simulink model "ExampleOrientationOnCar"  (Simulink 9.2)
settings: Solver=FixedStepDiscrete  StartTime=0.0  StopTime=inf  FixedStep=TIMESTEP  RelTol=1e-3  EnableMultiTasking=on
PostLoadFcn:
  | TIMESTEP = 0.001;
  | 
  | gCGHeight = 0.3545;            % height of the car body reference point above the ground
  | gLeftWheelBase = 3.105;      % distance between left front and rear axles
  | CG_OFFSET_FROM_NOSE = [-gLeftWheelBase/2, 0, gCGHeight];
libraries: simulink x6, rFproPhysicsLib x4
settings Model: Creator=enewton  LastModifiedBy=SeanKavanagh
settings OptimizationCC: ExpressionDepthLimit=2147483647  EfficientFloat2IntCast=on
settings DebuggingCC: SolverPrmCheckMsg=warning
settings RTWCC: SystemTargetFile=rfpro.tlc  MakeCommand="make_rtw OPTS=\"-DRUN_PHYSICS\""  TemplateMakefile=rfpro.tmf  Description=rFpro Target (Run Physics)  TargetLang=C++
settings STFCustomTargetCC: ModelReferenceCompliant=off  GeneratePreprocessorConditionals=Disable all  CombineOutputUpdateFcns=on  MatFileLogging=on  CPPClassGenCompliant=on  GRTInterface=off  SystemTargetFile=rfpro.tlc
settings GRTTargetCC: ModelReferenceCompliant=off  ParMdlRefBuildCompliant=off  CompOptLevelCompliant=off  ConcurrentExecutionCompliant=off  CombineOutputUpdateFcns=on  GRTInterface=off  UseToolchainInfoCompliant=off

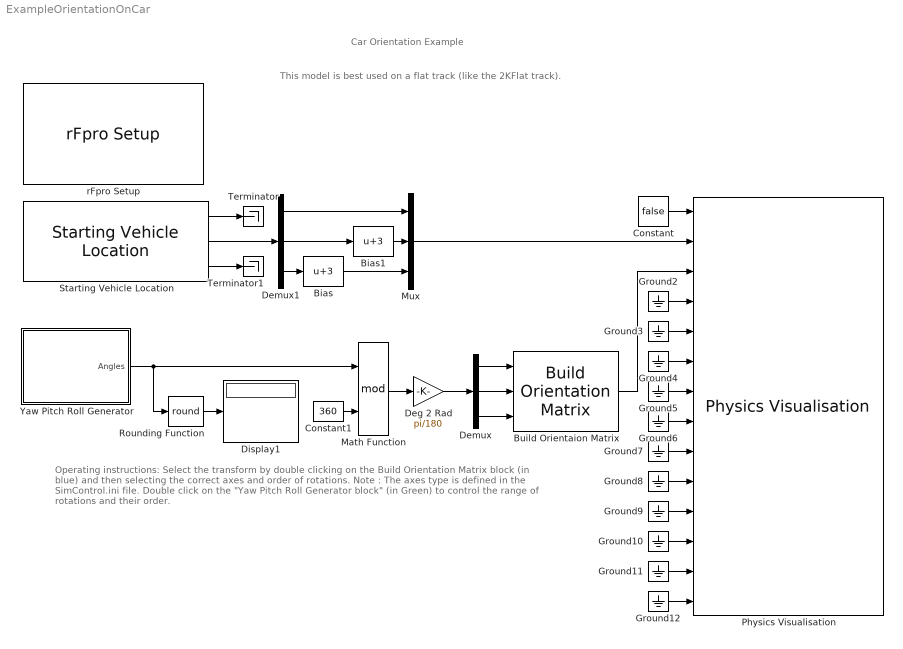
== system ExampleOrientationOnCar ==
  note: This model is best used on a flat track (like the 2KFlat track).
  note: Car Orientation Example
  note: Operating instructions:
      |
      | Select the transform by double clicking on the Build Orientation Matrix block (in blue)
      | and then selecting the correct axes and order of rotations.
      | Note : The axes type is defined in the SimControl.ini file.
      |
      | Double click on the "Yaw Pitch Roll Generator block" (in Green) to control the range
      | of rotations and their order.
  Bias : Bias  Bias=3
  Bias1 : Bias  Bias=3
  Build Orientaion Matrix : rFproPhysicsLib/Build Orientation Matrix  ISOAxes=on  YPROrder=on
  Constant : Constant  Value=false
  Constant1 : Constant  Value=360
  Deg 2 Rad : Gain  Gain=pi/180
  Demux : Demux  Outputs=3
  Demux1 : Demux  Outputs=3
  Display1 : Display
  Ground{2..12} (11 alike) : Ground
  Math Function : Math  Operator=mod  SaturateOnIntegerOverflow=on
  Mux : Mux  Inputs=3
  Physics Visualisation : rFproPhysicsLib/Physics Visualisation  PAR_SKIP_INTERNAL_PHYSICS=off  PAR_ACCEL_VALID=off  PAR_ROT_ACCEL_VALID=off  PAR_GEAR_VALID=off  PAR_RPM_VALID=off  PAR_INPUTS_VALID=on  PAR_STEER_TORQUE_VALID=on  PAR_HEADLIGHTS_ON_VALID=off  PAR_WHEEL_POS_VALID=off  PAR_WHEEL_ORI_VALID=off  PAR_TYRE_PARAMS_VALID=off  PAR_WHEEL_ROTATION_VALID=off  PAR_WHEEL_BRAKE_TEMP_VALID=off  PAR_WHEEL_TREAD_TEMP_VALID=off  PAR_WHEEL_AIR_TEMP_VALID=off  period=-1  offset=0  useReverseByteOrder=on  rFpro__platform=Remote Model - Default
  Rounding Function : Rounding  Operator=round
  Starting Vehicle Location : rFproPhysicsLib/Starting Vehicle Location  cg_offset=CG_OFFSET_FROM_NOSE  numPackets=1  rFpro__platform=Remote Model - Default
  Terminator : Terminator
  Terminator1 : Terminator
  Yaw Pitch Roll Generator : Subsystem  mask(Yaw, Pitch and Roll Generator){maxYaw=105, maxPitch=30, maxRoll=60, angleSpeed=1, YPR=on}
      mask prompts: maxYaw "Max Yaw (degrees)"; maxPitch "Max Pitch (degrees)"; maxRoll "Max Roll (degrees)"; angleSpeed "Speed"; YPR "Rotation order is YPR"
      mask help:
      | Enter the maximum values for the roll, pitch and yaw and the
      | output will run from zero to the maximum of each in turn,
      | holding the last value for the other angles.
      |
      | Speed scales how fast the angles change (default is 1).
      |
      | The order in which each is increased is set using the YPR checkbox.
  rFpro Setup : rFproPhysicsLib/rFpro Setup  platform=Remote Model - Default  stopOnSessionEnd=on  usePseudoRealtime=on  syncToRF=on  useReverseByteOrder=off  useRfTime=on  minIterations=4  maxIterations=1000  ipReceiveAddress='127.0.0.1'  ipReceivePort=11054  receiveSampleTime=-1  ipTransmitAddress='127.0.0.1'  ipTransmitPort=11052  transmitSampleTime=-1  pluginType=RUN_PHYSICS  sysTarget=xpctarget.tlc  templateMakeFile=xpc_default_tmf  makeCommand=make_rtw  buildDesc=xPC target
  wires:
  Constant/1 -> Physics Visualisation/1
  Ground2/1 -> Physics Visualisation/4
  Ground3/1 -> Physics Visualisation/5
  Ground4/1 -> Physics Visualisation/6
  Ground5/1 -> Physics Visualisation/7
  Ground6/1 -> Physics Visualisation/8
  Ground7/1 -> Physics Visualisation/9
  Ground8/1 -> Physics Visualisation/10
  Ground9/1 -> Physics Visualisation/11
  Ground10/1 -> Physics Visualisation/12
  Ground11/1 -> Physics Visualisation/13
  Ground12/1 -> Physics Visualisation/14
  Constant1/1 -> Math Function/2
  Math Function/1 -> Deg 2 Rad/1
  Starting Vehicle Location/1 -> Terminator/1
  Starting Vehicle Location/3 -> Terminator1/1
  Yaw Pitch Roll Generator/1(Angles) -> Math Function/1, Rounding Function/1
  Deg 2 Rad/1 -> Demux/1
  Mux/1 -> Physics Visualisation/2
  Starting Vehicle Location/2 -> Demux1/1
  Demux1/3 -> Bias/1
  Bias/1 -> Mux/3
  Demux1/2 -> Bias1/1
  Demux1/1 -> Mux/1
  Rounding Function/1 -> Display1/1
  Build Orientaion Matrix/1 -> Physics Visualisation/3
  Bias1/1 -> Mux/2
  Demux/1 -> Build Orientaion Matrix/1
  Demux/3 -> Build Orientaion Matrix/3
  Demux/2 -> Build Orientaion Matrix/2

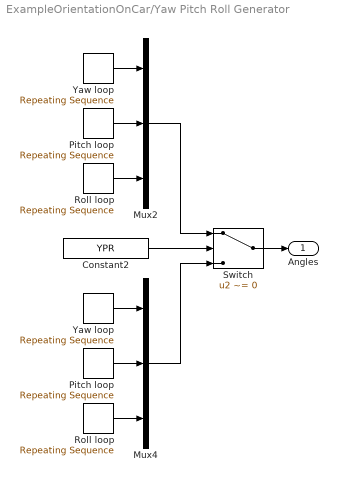
== system ExampleOrientationOnCar/Yaw Pitch Roll Generator ==
  Constant2 : Constant  Value=YPR
  Mux2 : Mux  Inputs=3
  Mux4 : Mux  Inputs=3
  Pitch loop : simulink/Sources/Repeating Sequence  rep_seq_t=(0:8) / angleSpeed  rep_seq_y=maxPitch * [0 0 1 1 1 1 0 0 0]
  "Pitch loop " : simulink/Sources/Repeating Sequence  rep_seq_t=(0:8) / angleSpeed  rep_seq_y=maxPitch * [0 0 0 1 1 0 0 0 0]
  Roll loop : simulink/Sources/Repeating Sequence  rep_seq_t=(0:8) / angleSpeed  rep_seq_y=maxRoll * [0 0 0 1 1 0 0 0 0]
  "Roll loop " : simulink/Sources/Repeating Sequence  rep_seq_t=(0:8) / angleSpeed  rep_seq_y=maxRoll * [0 0 1 1 1 1 0 0 0]
  Switch : Switch  Criteria=u2 ~= 0
  Yaw loop : simulink/Sources/Repeating Sequence  rep_seq_t=(0:8) / angleSpeed  rep_seq_y=maxYaw * [0 1 1 1 1 1 1 0 0]
  "Yaw loop " : simulink/Sources/Repeating Sequence  rep_seq_t=(0:8) / angleSpeed  rep_seq_y=maxYaw * [0 1 1 1 1 1 1 0 0]
  Angles : Outport
  wires:
  Switch/1 -> Angles/1
  Yaw loop/1 -> Mux2/1
  Pitch loop/1 -> Mux2/2
  Roll loop/1 -> Mux2/3
  "Yaw loop "/1 -> Mux4/1
  "Pitch loop "/1 -> Mux4/2
  "Roll loop "/1 -> Mux4/3
  Mux2/1 -> Switch/1
  Mux4/1 -> Switch/3
  Constant2/1 -> Switch/2
